simulink model "lqr_method"  (R2023a)
settings: Solver=VariableStepAuto  StartTime=0.0  StopTime=10.0  RelTol=1e-3
values from neighbouring files (symbols this model uses):
  A_pitch = [0,1;0,sin(beta)/Iyy*(N^2/R+c)*(-2*sin(beta)-Iyy/(Iw_pitch*sin(beta)))]    [main.m]
  A_roll = [0,1;0,sin(beta)/Ixx*(N^2/R+c)*(-2*sin(beta)-Ixx/(Iw_roll*sin(beta)))]    [main.m]
  B_pitch = [0;sin(beta)/Iyy*N/R]    [main.m]
  B_roll = [0;sin(beta)/Ixx*N/R]    [main.m]
  beta = 63.4*pi/180    (= 1.10653874576)    [lqr_meth.m]    (also in main.m = deg2rad(63.4))
  degree_p = 30    [main.m]
  Iw_pitch = T / (2 * Omega_dot * sin(beta))    [Compute_pitch.m]    (also in main.m = Iw_pitch * 50)
  Iw_roll = T/(2*Omega_dot*sin(beta))    [Compute_roll.m]    (also in main.m = Iw_roll * 50)
  Ixx = 10^6    (= 1000000)    [main.m]
  Iyy = 10^6    (= 1000000)    [main.m]
  K_pitch = lqr(A_pitch,B_pitch,Q_pitch,R_pitch)    [main.m]
  K_roll = lqr(A_roll,B_roll,Q_roll,R_roll)    [main.m]
  N = 169.8485    [main.m]
  R = 1/i    [FindQR_minPower.m]    (also in FindQR_test.m; lqr_meth.m; main.m = 0.101)
  theta_roll_final = deg2rad(90)    [main.m]
settings Model: Creator=Home  LastModifiedBy=Home

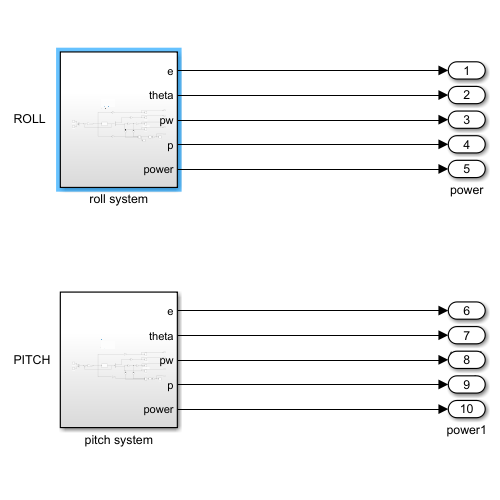
[thumbnail: Simulink's stored preview of the top-level diagram]
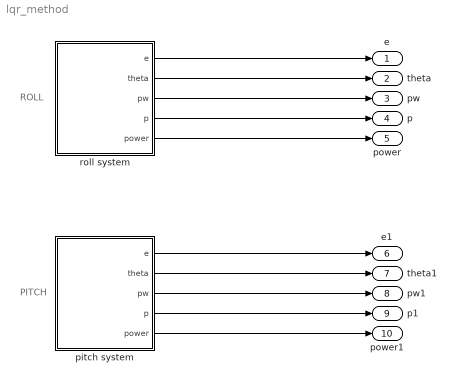
== system lqr_method ==
  note: ROLL
  note: PITCH
  pitch system : Subsystem
  roll system : Subsystem
  e : Outport
  theta : Outport  Port=2
  pw : Outport  Port=3
  p : Outport  Port=4
  power : Outport  Port=5
  e1 : Outport  Port=6
  theta1 : Outport  Port=7
  pw1 : Outport  Port=8
  p1 : Outport  Port=9
  power1 : Outport  Port=10
  wires:
  roll system/2(theta) -> theta/1
  roll system/3(pw) -> pw/1
  roll system/1(e) -> e/1
  roll system/5(power) -> power/1
  roll system/4(p) -> p/1
  pitch system/3(pw) -> pw1/1
  pitch system/2(theta) -> theta1/1
  pitch system/1(e) -> e1/1
  pitch system/5(power) -> power1/1
  pitch system/4(p) -> p1/1

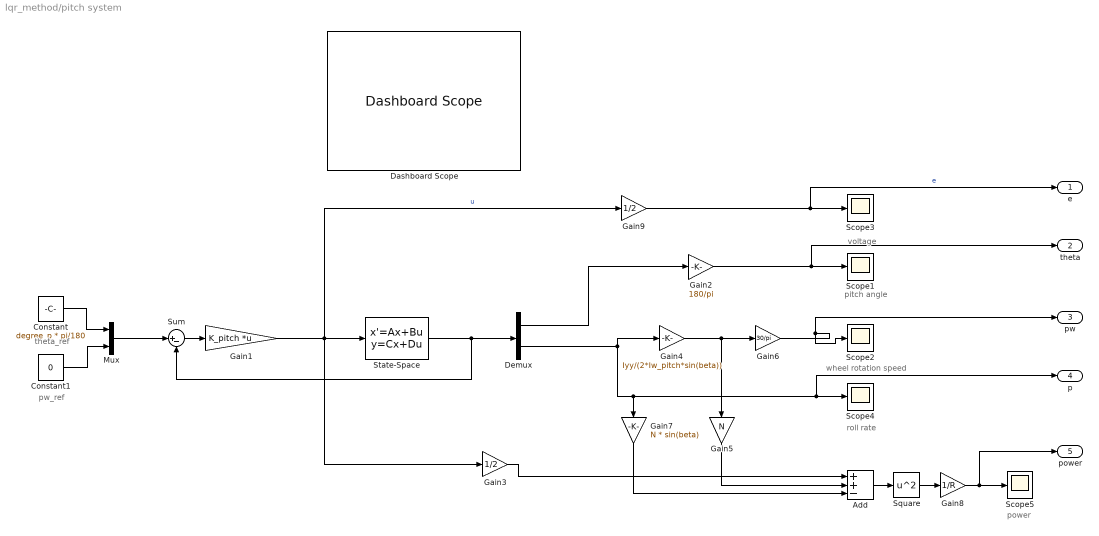
== system lqr_method/pitch system ==
  note: wheel rotation speed
  note: power
  note: pitch angle
  note: theta_ref
  note: voltage
  note: pw_ref
  note: roll rate
  Add : Sum  Inputs=++-
  Constant : Constant  Value=degree_p * pi/180
  Constant1 : Constant  Value=0
  Dashboard Scope : DashboardScope
  Demux : Demux  Outputs=2
  Gain1 : Gain  Gain=K_pitch  Multiplication=Matrix(K*u) (u vector)
  Gain2 : Gain  Gain=180/pi
  Gain3 : Gain  Gain=1/2
  Gain4 : Gain  Gain=Iyy/(2*Iw_pitch*sin(beta))
  Gain5 : Gain  Gain=N
  Gain6 : Gain  Gain=30/pi
  Gain7 : Gain  Gain=N * sin(beta)
  Gain8 : Gain  Gain=1/R
  Gain9 : Gain  Gain=1/2
  Mux : Mux  Inputs=2
  Scope{1..5} (5 alike) : Scope
  Square : Math  Operator=square
  State-Space : StateSpace  A=A_pitch  B=B_pitch  C=eye(2)  D=[0;0]  InitialCondition=[0 0]
  Sum : Sum  Inputs=|+-
  e : Outport
  theta : Outport  Port=2
  pw : Outport  Port=3
  p : Outport  Port=4
  power : Outport  Port=5
  wires:
  Gain8/1 -> power/1, Scope5/1
  Gain6/1 -> Scope2/1, pw/1
  Gain5/1 -> Add/2
  Square/1 -> Gain8/1
  Gain3/1 -> Add/1
  Gain7/1 -> Add/3
  Gain2/1 -> theta/1, Scope1/1
  Gain1/1 -> Gain3/1, Gain9/1, State-Space/1  "u"
  Demux/1 -> Gain2/1
  State-Space/1 -> Sum/2, Demux/1
  Gain4/1 -> Gain5/1, Gain6/1
  Mux/1 -> Sum/1
  Demux/2 -> Gain7/1, p/1, Scope4/1, Gain4/1
  Constant1/1 -> Mux/2
  Sum/1 -> Gain1/1
  Add/1 -> Square/1
  Constant/1 -> Mux/1
  Gain9/1 -> e/1, Scope3/1  "e"

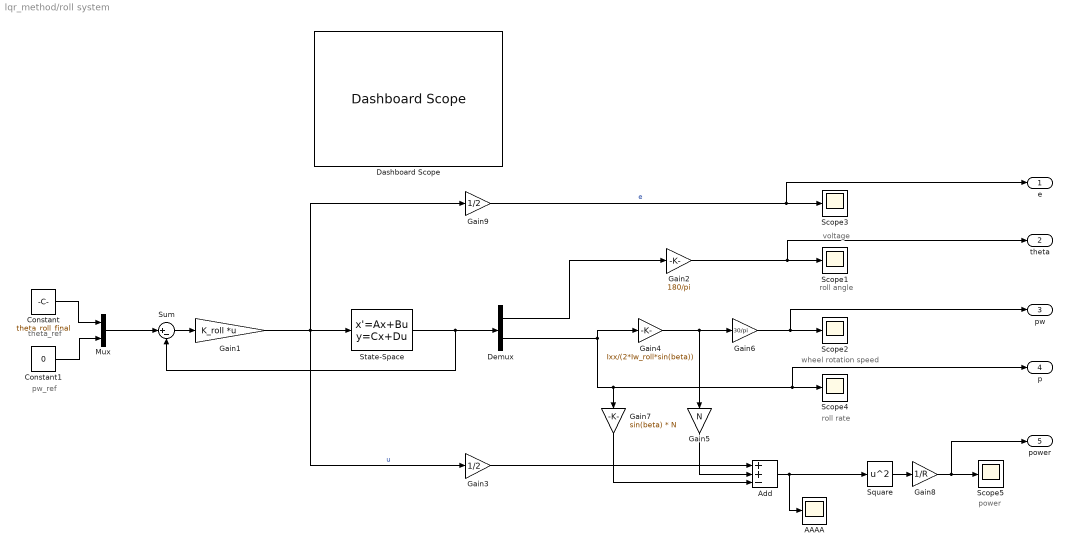
== system lqr_method/roll system ==
  note: wheel rotation speed
  note: power
  note: roll angle
  note: theta_ref
  note: voltage
  note: pw_ref
  note: roll rate
  AAAA : Scope
  Add : Sum  Inputs=++-
  Constant : Constant  Value=theta_roll_final
  Constant1 : Constant  Value=0
  Dashboard Scope : DashboardScope
  Demux : Demux  Outputs=2
  Gain1 : Gain  Gain=K_roll  Multiplication=Matrix(K*u) (u vector)
  Gain2 : Gain  Gain=180/pi
  Gain3 : Gain  Gain=1/2
  Gain4 : Gain  Gain=Ixx/(2*Iw_roll*sin(beta))
  Gain5 : Gain  Gain=N
  Gain6 : Gain  Gain=30/pi
  Gain7 : Gain  Gain=sin(beta) * N
  Gain8 : Gain  Gain=1/R
  Gain9 : Gain  Gain=1/2
  Mux : Mux  Inputs=2
  Scope{1..5} (5 alike) : Scope
  Square : Math  Operator=square
  State-Space : StateSpace  A=A_roll  B=B_roll  C=eye(2)  D=[0;0]  InitialCondition=[0 0]
  Sum : Sum  Inputs=|+-
  e : Outport
  theta : Outport  Port=2
  pw : Outport  Port=3
  p : Outport  Port=4
  power : Outport  Port=5
  wires:
  Gain8/1 -> power/1, Scope5/1
  Gain5/1 -> Add/2
  Square/1 -> Gain8/1
  Gain3/1 -> Add/1
  Gain7/1 -> Add/3
  Gain2/1 -> theta/1, Scope1/1
  Gain1/1 -> Gain3/1, Gain9/1, State-Space/1  "u"
  Demux/1 -> Gain2/1
  State-Space/1 -> Sum/2, Demux/1
  Gain4/1 -> Gain5/1, Gain6/1
  Mux/1 -> Sum/1
  Demux/2 -> Gain7/1, p/1, Scope4/1, Gain4/1
  Constant1/1 -> Mux/2
  Sum/1 -> Gain1/1
  Add/1 -> AAAA/1, Square/1
  Constant/1 -> Mux/1
  Gain9/1 -> e/1, Scope3/1  "e"
  Gain6/1 -> pw/1, Scope2/1
